simulink library "magnetometer_lib"  (R2016b)
settings: Solver=VariableStepAuto  StartTime=0.0  StopTime=10.0  RelTol=1e-3
libraries: dspmathops x2, aerolibutil x1
settings Model: Creator=Taylor  LastModifiedBy=Taylor
settings OptimizationCC: LifeSpan=inf
settings DebuggingCC: SFExecutionAtInitializationDiag=none

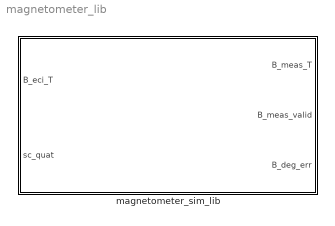
== system magnetometer_lib ==
  magnetometer_sim_lib : Subsystem  mask{seed_x=4, seed_y=5, seed_z=6}
      mask prompts: seed_x "Seed the x-axis random noise generator"; seed_y "seed the y-axis random noise generator"; seed_z "Seed the z-axis random noise generator"
      mask TypeOptions seed_x: gaussian_error_vector/Random Number2/Seed
      mask TypeOptions seed_y: gaussian_error_vector/Random Number3/Seed
      mask TypeOptions seed_z: gaussian_error_vector/Random Number4/Seed

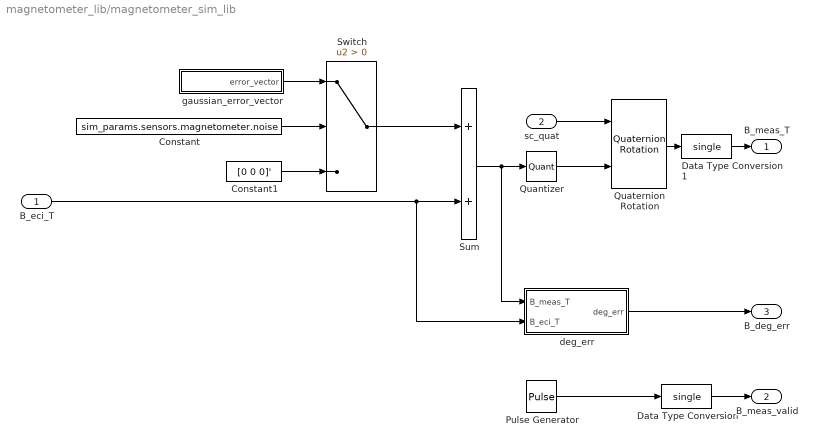
== system magnetometer_lib/magnetometer_sim_lib ==
  B_eci_T : Inport
  sc_quat : Inport  Port=2
  Constant : Constant  Value=sim_params.sensors.magnetometer.noise
  Constant1 : Constant  Value=[0 0 0]'
  Data Type Conversion : DataTypeConversion  OutDataTypeStr=single
  Data Type Conversion1 : DataTypeConversion  OutDataTypeStr=single
  Pulse Generator : DiscretePulseGenerator  PulseType=Time based  Period=10  PulseWidth=sim_params.sensors.magnetometer.valid_pct
  Quantizer : Quantizer  QuantizationInterval=sim_params.sensors.magnetometer.resolution
  Quaternion Rotation : aerolibutil/Quaternion Rotation
  Sum : Sum
  Switch : Switch  Criteria=u2 > Threshold
  deg_err : Subsystem
  gaussian_error_vector : Subsystem
  B_meas_T : Outport
  B_meas_valid : Outport  Port=2
  B_deg_err : Outport  Port=3
  wires:
  Quaternion Rotation/1 -> Data Type Conversion1/1
  sc_quat/1 -> Quaternion Rotation/1
  Pulse Generator/1 -> Data Type Conversion/1
  Switch/1 -> Sum/1
  Constant/1 -> Switch/2
  Sum/1 -> Quantizer/1, deg_err/1(B_meas_T)
  Constant1/1 -> Switch/3
  gaussian_error_vector/1(error_vector) -> Switch/1
  B_eci_T/1 -> deg_err/2(B_eci_T), Sum/2
  deg_err/1(deg_err) -> B_deg_err/1
  Quantizer/1 -> Quaternion Rotation/2
  Data Type Conversion/1 -> B_meas_valid/1
  Data Type Conversion1/1 -> B_meas_T/1

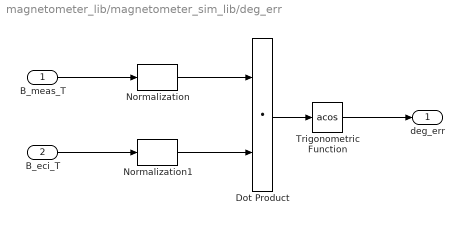
== system magnetometer_lib/magnetometer_sim_lib/deg_err ==
  B_meas_T : Inport
  B_eci_T : Inport  Port=2
  Dot Product : DotProduct  InputSameDT=on  OutDataTypeStr=Inherit: Inherit via internal rule
  Normalization : dspmathops/Normalization  NormType=2-norm  Bias=1e-10  NormOver=Each column  Dimension=1  outputDataTypeStr=Inherit: Same as product output  outputLastDataTypeStr=Inherit: Same as product output  outputMin=[]  outputMax=[]  accumDataTypeStr=Inherit: Same as product output  accumLastDataTypeStr=Inherit: Same as product output  roundingMode=Floor  overflowMode=off
  Normalization1 : dspmathops/Normalization  NormType=2-norm  Bias=1e-10  NormOver=Each column  Dimension=1  outputDataTypeStr=Inherit: Same as product output  outputLastDataTypeStr=Inherit: Same as product output  outputMin=[]  outputMax=[]  accumDataTypeStr=Inherit: Same as product output  accumLastDataTypeStr=Inherit: Same as product output  roundingMode=Floor  overflowMode=off
  Trigonometric Function : Trigonometry  Operator=acos
  deg_err : Outport
  wires:
  B_meas_T/1 -> Normalization/1
  Normalization/1 -> Dot Product/1
  B_eci_T/1 -> Normalization1/1
  Dot Product/1 -> Trigonometric Function/1
  Trigonometric Function/1 -> deg_err/1
  Normalization1/1 -> Dot Product/2

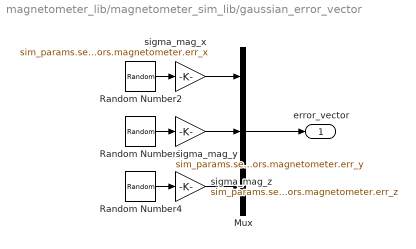
== system magnetometer_lib/magnetometer_sim_lib/gaussian_error_vector ==
  Mux : Mux  Inputs=3
  Random Number2 : RandomNumber  Seed=seed_x  SampleTime=sim_params.sensors.magnetometer.sample_time_s
  Random Number3 : RandomNumber  Seed=seed_y  SampleTime=sim_params.sensors.magnetometer.sample_time_s
  Random Number4 : RandomNumber  Seed=seed_z  SampleTime=sim_params.sensors.magnetometer.sample_time_s
  sigma_mag_x : Gain  Gain=sim_params.sensors.magnetometer.err_x
  sigma_mag_y : Gain  Gain=sim_params.sensors.magnetometer.err_y
  sigma_mag_z : Gain  Gain=sim_params.sensors.magnetometer.err_z
  error_vector : Outport
  wires:
  Random Number2/1 -> sigma_mag_x/1
  Random Number4/1 -> sigma_mag_z/1
  Random Number3/1 -> sigma_mag_y/1
  sigma_mag_x/1 -> Mux/1
  sigma_mag_y/1 -> Mux/2
  Mux/1 -> error_vector/1
  sigma_mag_z/1 -> Mux/3
